simulink model "HDLBitShift"  (R2024a)
settings: Solver=FixedStepDiscrete  StartTime=0.0  StopTime=20/125e6  RelTol=1e-3
libraries: hdlsllib x1
settings Model: DataTypeOverride=Off  Creator=cotti  LastModifiedBy=cotti
settings OptimizationCC: BlockReduction=off  ConditionallyExecuteInputs=off  DefaultParameterBehavior=Inlined  InheritOutputTypeSmallerThanSingle=on
settings DebuggingCC: AlgebraicLoopMsg=error  ArtificialAlgebraicLoopMsg=error  SingleTaskRateTransMsg=error  UnconnectedInputMsg=warning  UnconnectedOutputMsg=warning  UnconnectedLineMsg=warning
settings HardwareCC: ProdBitPerPointer=32  ProdBitPerSizeT=32  ProdBitPerPtrDiffT=32  ProdLargestAtomicFloat=None  ProdIntDivRoundTo=Undefined  ProdEndianess=Unspecified  ProdWordSize=32  ProdHWDeviceType=ASIC/FPGA->ASIC/FPGA  TargetBitPerLong=64  TargetBitPerPointer=64  TargetBitPerSizeT=64  TargetBitPerPtrDiffT=64  TargetLongLongMode=on  TargetIntDivRoundTo=Zero  TargetEndianess=LittleEndian  TargetWordSize=64  TargetHWDeviceType=Custom Processor->MATLAB Host Computer  ProdEqTarget=off

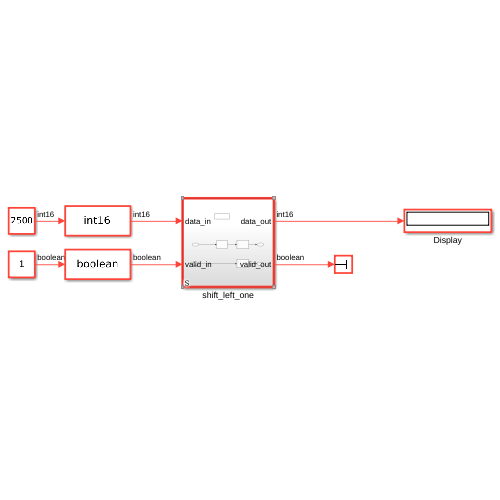
[thumbnail: Simulink's stored preview of the top-level diagram]
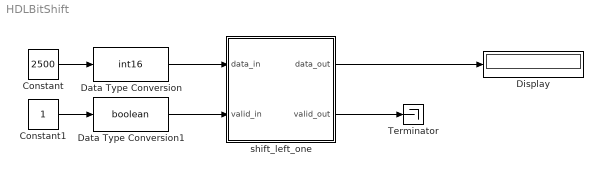
== system HDLBitShift ==
  Constant : Constant  Value=2500  OutDataTypeStr=int16  SampleTime=1/125e6
  Constant1 : Constant  OutDataTypeStr=boolean  SampleTime=1/125e6
  Data Type Conversion : DataTypeConversion  OutDataTypeStr=int16  SaturateOnIntegerOverflow=off  RndMeth=Floor
  Data Type Conversion1 : DataTypeConversion  OutDataTypeStr=boolean  SaturateOnIntegerOverflow=off  RndMeth=Floor
  Display : Display
  Terminator : Terminator
  shift_left_one : Subsystem  TreatAsAtomicUnit=on
  wires:
  Constant/1 -> Data Type Conversion/1
  Data Type Conversion/1 -> shift_left_one/1(data_in)
  shift_left_one/2(valid_out) -> Terminator/1
  Constant1/1 -> Data Type Conversion1/1
  Data Type Conversion1/1 -> shift_left_one/2(valid_in)
  shift_left_one/1(data_out) -> Display/1

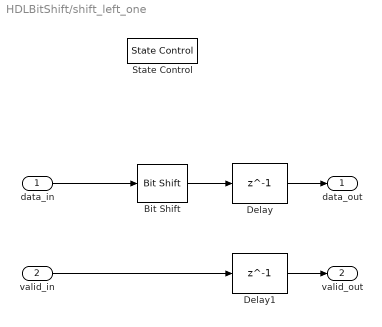
== system HDLBitShift/shift_left_one ==
  data_in : Inport
  valid_in : Inport  Port=2
  Bit Shift : hdlsllib/Logic and Bit Operations/Bit Shift  mode=Shift Left Logical  N=1
  Delay : Delay  DelayLength=1  InitialCondition=0  UseCircularBuffer=on
  Delay1 : Delay  DelayLength=1  InitialCondition=0  UseCircularBuffer=on
  State Control : StateControl  StateControl=Synchronous
  data_out : Outport
  valid_out : Outport  Port=2
  wires:
  data_in/1 -> Bit Shift/1
  Bit Shift/1 -> Delay/1
  Delay/1 -> data_out/1
  Delay1/1 -> valid_out/1
  valid_in/1 -> Delay1/1
